simulink model "Simulator_Blockset"  (R2017b)
settings: Solver=VariableStepAuto  StartTime=0.0  StopTime=300  RelTol=1e-3  EnableMultiTasking=on
InitFcn:
  | Simulator_Init;
StopFcn:
  | % xia_out
values from neighbouring files (symbols this model uses):
  CC0 = 0    [Simulator_Init.m]
  CC_alpha = 0    [Simulator_Init.m]
  CC_beta = num(8,1)    [Simulator_Init.m]    (also in lat_eig.m = STB_LATin.DRVs.CC_beta)
  CC_dr = num(8,13)    [Simulator_Init.m]
  CC_p = num(8,4)    [Simulator_Init.m]
  CC_q = 0    [Simulator_Init.m]
  CC_r = num(8,5)    [Simulator_Init.m]
  CD0 = num(11,2)    [Simulator_Init.m]    (also in VLM2FG.m = Results.state(1,1).STC.friction.CD0; lat_chr.m = FILE.M_SDRV.state(1,1).STC.CD-FILE.M_SDRV.state(1,1).STC.CDi)
  CD_alpha = num(5,2)    [Simulator_Init.m]    (also in long_eig.m = results.CD_alpha)
  CD_alpha_dot = num(5,8)    [Simulator_Init.m]    (also in long_eig.m = 0)
  CD_beta = 0    [Simulator_Init.m]
  CD_dr = 0    [Simulator_Init.m]
  CD_p = num(5,17)    [Simulator_Init.m]
  CD_q = num(5,12)    [Simulator_Init.m]    (also in long_eig.m = results.CD_Q)
  CD_r = 0    [Simulator_Init.m]
  CL0 = num(11,1)    [Simulator_Init.m]
  CL_alpha = num(5,1)    [Simulator_Init.m]    (also in long_eig.m = results.CL_alpha; long_gfix.m = Mfile(i).M_SDRV.CL_alpha)
  CL_alpha_dot = num(5,7)    [Simulator_Init.m]    (also in long_eig.m = 0)
  CL_beta = num(5,16)    [Simulator_Init.m]
  CL_p = 0    [Simulator_Init.m]
  CL_q = num(5,10)    [Simulator_Init.m]    (also in long_eig.m = results.CL_Q)
  CL_r = 0    [Simulator_Init.m]
  Clm0 = 0    [Simulator_Init.m]
  Clm_alpha = 0    [Simulator_Init.m]
  Clm_beta = num(8,2)    [Simulator_Init.m]    (also in lat_eig.m = -0.074)
  Clm_da = num(8,11)    [Simulator_Init.m]
  Clm_dr = num(8,14)    [Simulator_Init.m]
  Clm_p = num(8,6)    [Simulator_Init.m]
  Clm_q = 0    [Simulator_Init.m]
  Clm_r = num(8,8)    [Simulator_Init.m]
  Cmm0 = 0    [Simulator_Init.m]
  Cmm_alpha = num(5,3)    [Simulator_Init.m]    (also in long_eig.m = results.CMm_alpha)
  Cmm_alpha_dot = num(5,9)    [Simulator_Init.m]    (also in long_eig.m = 0)
  Cmm_beta = 0    [Simulator_Init.m]
  Cmm_de = num(5,15)    [Simulator_Init.m]
  Cmm_p = num(8,19)    [Simulator_Init.m]
  Cmm_q = num(5,11)    [Simulator_Init.m]    (also in long_eig.m = results.CMm_Q)
  Cmm_r = 0    [Simulator_Init.m]
  Cnm0 = 0    [Simulator_Init.m]
  Cnm_alpha = 0    [Simulator_Init.m]
  Cnm_beta = num(8,3)    [Simulator_Init.m]    (also in lat_eig.m = 0.0701)
  Cnm_dr = num(8,15)    [Simulator_Init.m]
  Cnm_p = num(8,7)    [Simulator_Init.m]
  Cnm_q = 0    [Simulator_Init.m]
  Cnm_r = num(8,9)    [Simulator_Init.m]
  Engine = Ctrl.ENG    [Simulator_Init.m]
  F = double(F)    [PHD_paracamber.m]
  q = 0.5*state.rho*state.AS^2    [coeff_create3.m]    (also in coeff_hinge.m; lat_eig.m = 0.5*rho*V^2; long_eig.m = 0.5*rho*V^2; long_gfix.m = .5*allstate.rho*allstate.AS0(j)^2)
  uaero0 = [0 0 0 0]    [Simulator_Init.m]
undefined symbols (not defined in the file or in its folder): Earth, Light, MIL, model, WGS84
libraries: aerolibfltsims x3, aerolibadynsys x2, aerolibwind2 x2, aerolibanimutils x2, aerolibconvert2 x2, shared6dof x1, instrumentlib x1, sharedutil x1, aerolibasang x1, simulink_extras x1, aerolibatmos2 x1, aerolibobsolete x1
CloseFcn:
  | clear all;
settings Model: Creator=mc  LastModifiedBy=SONG
settings DataIOCC: LimitDataPoints=on  SaveFormat=Array
settings OptimizationCC: LifeSpan=inf
settings DebuggingCC: SolverPrmCheckMsg=warning  AllowSymbolicDim=off  SFUnexpectedBacktrackingDiag=warning  SFNoUnconditionalDefaultTransitionDiag=warning  SFExecutionAtInitializationDiag=none
settings HardwareCC: ProdBitPerPointer=32  ProdBitPerSizeT=32  ProdBitPerPtrDiffT=32  ProdLargestAtomicFloat=None  ProdIntDivRoundTo=Undefined  ProdEndianess=Unspecified  ProdWordSize=32  ProdHWDeviceType=32-bit Generic
settings ModelReferenceCC: PropagateSignalLabelsOutOfModel=off
settings CodeAppCC: StateflowObjectComments=on
settings GRTTargetCC: TargetLangStandard=C89/C90 (ANSI)  GeneratePreprocessorConditionals=Disable all
settings ConfigComp: CovMetricSettings=dw  CovHtmlReporting=on  CovSaveCumulativeToWorkspaceVar=on  CovSaveSingleToWorkspaceVar=on  CovExternalEMLEnable=off  CovSFcnEnable=off

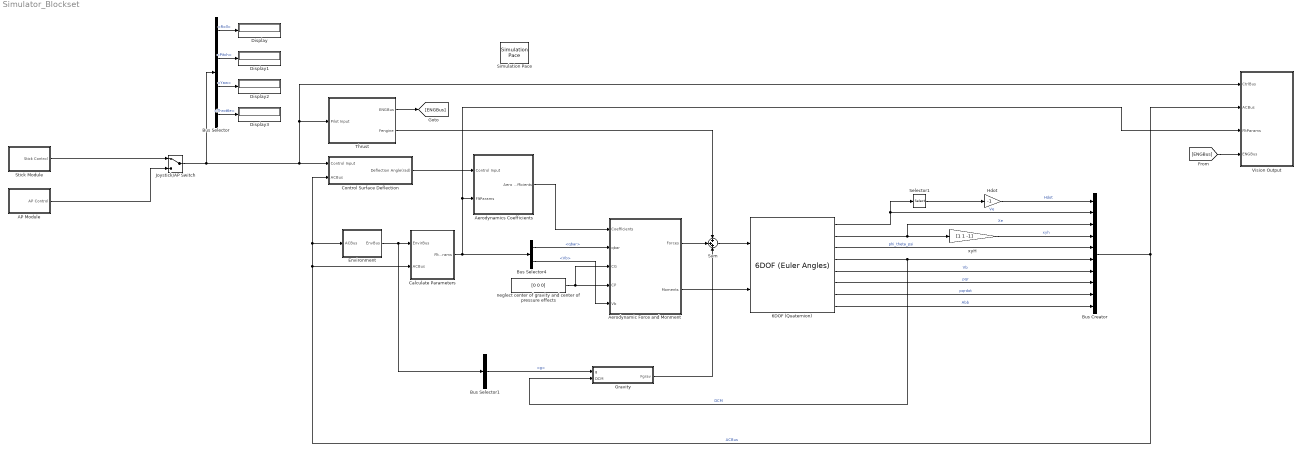
== system Simulator_Blockset ==
  6DOF (Quaternion) : shared6dof/6DOF (Euler Angles)  units=Metric (MKS)  mtype=Fixed  rep=Quaternion  xme_0=xme_0  Vm_0=[model.init.U model.init.V model.init.W]  eul_0=[model.init.roll, model.init.pitch, model.init.yaw]  pm_0=[model.init.P, model.init.Q, model.init.R]  mass_0=model.mass  mass_e=0  mass_f=0  inertia=[model.Ix -model.Ixy -model.Ixz; -model.Iyx model.Iy -model.Iyz; -model.Izx -model.Izy model.Iz]  inertia_e=eye(3)  inertia_f=eye(3)  k_quat=1.0  vre_flag=on  abi_flag=off
      settings: SourceProductBaseCode=AE
  AP Module : Subsystem
  Aerodynamic Force and Monment : Subsystem
  Aerodynamics Coefficients : Subsystem
  Bus Creator : BusCreator  Inputs=10
  Bus Selector : BusSelector  OutputSignals=Roll,Pitch,Yaw,Throttle
  Bus Selector1 : BusSelector  OutputSignals=g
  Bus Selector4 : BusSelector  OutputSignals=qbar,Vb
  Calculate Parameters : Subsystem
  Control Surface Deflection : Subsystem  mask{PitchUp_Lim=20, PitchDown_Lim=10, Roll_Lim=20, Yaw_Lim=20}
      mask prompts: PitchUp_Lim "Pitch Up Limit (Deg)"; PitchDown_Lim "Pitch Down Limit (Deg)"; Roll_Lim "Roll Limit (Deg)"; Yaw_Lim "Yaw Limit (Deg)"
      mask DialogControl ParameterGroupVar Prompt: Deflection Limits
  Display{,1..3} (4 alike) : Display
  Environment : Subsystem
  "Gravity " : Subsystem
  Hdot : Gain  Gain=-1  SaturateOnIntegerOverflow=on  OutDataTypeStr=Inherit: Same as input  ParamDataTypeStr=Inherit: Same as input
  Joystick/AP Switch : ManualSwitch
  Selector1 : Selector  IndexMode=Zero-based  InputPortWidth=3  IndexOptions=Index vector (dialog)  Indices=2  OutputSizes=1
  Simulation Pace : aerolibanimutils/Simulation Pace  SimulationPace=1  SleepMode=MATLAB Thread  OutputPaceError=off  SampleTime=1/50
      settings: AttributesFormatString=%<SimulationPace> sec/sec
  Stick Module : Subsystem
  Sum : Sum  Inputs=+++  SaturateOnIntegerOverflow=on  InputSameDT=on  OutDataTypeStr=Inherit: Same as first input
  Thrust : Subsystem
  Vision Output : Subsystem
  neglect center of gravity and center of pressure effects : Constant  Value=[0 0 0]
  xyH : Gain  Gain=[1 1 -1]  SaturateOnIntegerOverflow=on  OutDataTypeStr=Inherit: Same as input  ParamDataTypeStr=Inherit: Same as input
  wires:
  Hdot/1 -> Bus Creator/1  "Hdot"
  xyH/1 -> Bus Creator/4  "xyh"
  6DOF (Quaternion)/6 -> Bus Creator/8  "pqr"
  6DOF (Quaternion)/5 -> Bus Creator/7  "Vb"
  Aerodynamics Coefficients/1(Aero Coefficients) -> Aerodynamic Force and Monment/1(Coefficients)
  6DOF (Quaternion)/1 -> Selector1/1, Bus Creator/2  "Ve"
  Selector1/1 -> Hdot/1
  Environment/1(EnvBus) -> Bus Selector1/1, Calculate Parameters/1(EnvirBus)
  neglect center of gravity and center of pressure effects/1 -> Aerodynamic Force and Monment/3(CG), Aerodynamic Force and Monment/4(CP)
  Aerodynamic Force and Monment/2(Moments) -> 6DOF (Quaternion)/2
  6DOF (Quaternion)/7 -> Bus Creator/9  "pqrdot"
  6DOF (Quaternion)/3 -> Bus Creator/5  "phi_theta_psi"
  6DOF (Quaternion)/4 -> "Gravity "/2(DCM), Bus Creator/6  "DCM"
  6DOF (Quaternion)/2 -> Bus Creator/3, xyH/1  "Xe"
  Bus Selector4/1 -> Aerodynamic Force and Monment/2(qbar)  "<qbar>"
  Sum/1 -> 6DOF (Quaternion)/1
  "Gravity "/1(Fgrav) -> Sum/3
  Aerodynamic Force and Monment/1(Forces) -> Sum/2
  Bus Creator/1 -> Environment/1(ACBus), Control Surface Deflection/2(ACBus), Calculate Parameters/2(ACBus), Vision Output/2(ACBus)  "ACBus"
  Thrust/2(Fengine) -> Sum/1
  Calculate Parameters/1(FltParams) -> Vision Output/3(FltParams), Aerodynamics Coefficients/2(FltParams), Bus Selector4/1
  Bus Selector4/2 -> Aerodynamic Force and Monment/5(Vb)  "<Vb>"
  Bus Selector1/1 -> "Gravity "/1(g)  "<g>"
  Control Surface Deflection/1(Deflection Angle(rad)) -> Aerodynamics Coefficients/1(Control Input)
  Joystick/AP Switch/1 -> Bus Selector/1, Vision Output/1(CtrlBus), Thrust/1(Pilot Input), Control Surface Deflection/1(Control Input)
  Stick Module/1(Stick Control) -> Joystick/AP Switch/1
  6DOF (Quaternion)/8 -> Bus Creator/10  "Abb"
  AP Module/1(AP Control) -> Joystick/AP Switch/2
  Thrust/1(ENGBus) -> [ENGBus]
  [ENGBus] -> Vision Output/4(ENGBus)
  Bus Selector/4 -> Display3/1  "<Throttle>"
  Bus Selector/2 -> Display1/1  "<Pitch>"
  Bus Selector/1 -> Display/1  "<Roll>"
  Bus Selector/3 -> Display2/1  "<Yaw>"

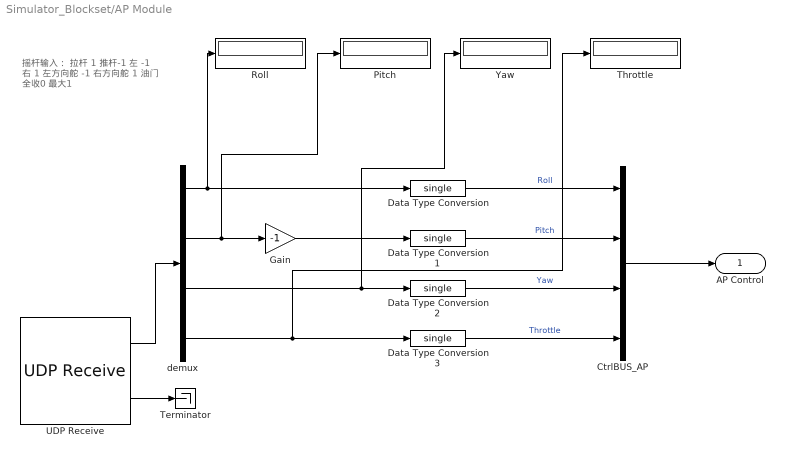
== system Simulator_Blockset/AP Module ==
  note: 摇杆输入：
      | 拉杆 1   推杆-1
      | 左   -1	右 1
      | 左方向舵 -1	右方向舵 1
      | 油门 全收0	最大1
  "CtrlBUS_AP " : BusCreator  Inputs=4
  Data Type Conversion{,1..3} (4 alike) : DataTypeConversion  OutDataTypeStr=single
  Gain : Gain  Gain=-1
  "Pitch " : Display
  Roll : Display
  Terminator : Terminator
  Throttle : Display
  UDP Receive : instrumentlib/UDP Receive  Host=127.0.0.1  Port=5500  LocalPort=49000  DataSize="[1  4]"  EnableBlockingMode=off  Timeout=10  SampleTime=-1  DataType=double  ByteOrder=BigEndian
      settings: SourceProductName=Instrument Control Toolbox
  Yaw : Display
  demux : Demux
  AP Control : Outport
  wires:
  demux/1 -> Roll/1, Data Type Conversion/1
  UDP Receive/2 -> Terminator/1
  UDP Receive/1 -> demux/1
  demux/3 -> Yaw/1, Data Type Conversion2/1
  demux/4 -> Throttle/1, Data Type Conversion3/1
  Data Type Conversion/1 -> "CtrlBUS_AP "/1  "Roll"
  Data Type Conversion1/1 -> "CtrlBUS_AP "/2  "Pitch"
  Data Type Conversion2/1 -> "CtrlBUS_AP "/3  "Yaw"
  Data Type Conversion3/1 -> "CtrlBUS_AP "/4  "Throttle"
  "CtrlBUS_AP "/1 -> AP Control/1
  demux/2 -> "Pitch "/1, Gain/1
  Gain/1 -> Data Type Conversion1/1

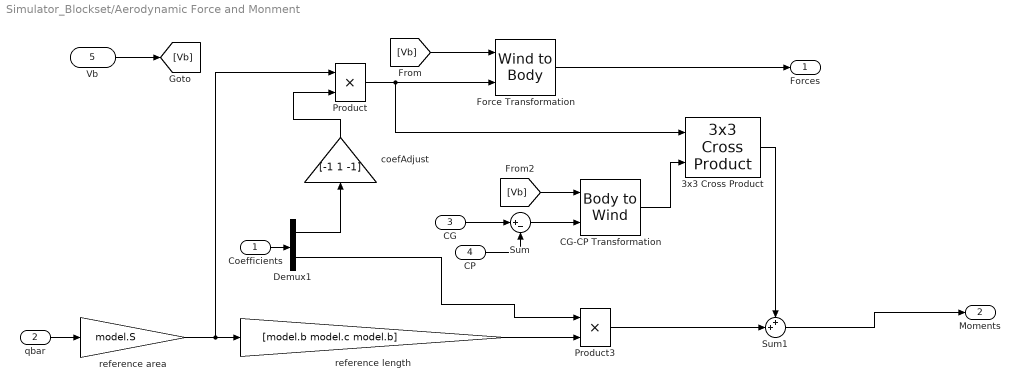
== system Simulator_Blockset/Aerodynamic Force and Monment ==
  Coefficients : Inport
  qbar : Inport  Port=2
  CG : Inport  Port=3
  CP : Inport  Port=4
  Vb : Inport  Port=5
  3x3 Cross Product : sharedutil/3x3 Cross Product
      settings: SourceProductBaseCode=AE
  CG-CP Transformation : aerolibadynsys/Body to Wind  SystemSampleTime=-1
      settings: SourceProductName=Aerospace Blockset  SourceProductBaseCode=AE
  Demux1 : Demux  Outputs=[3,3]
  Force Transformation : aerolibadynsys/Wind to Body  SystemSampleTime=-1
      settings: SourceProductName=Aerospace Blockset  SourceProductBaseCode=AE
  Product : Product  SaturateOnIntegerOverflow=on  InputSameDT=on  OutDataTypeStr=Inherit: Same as first input
  Product3 : Product  SaturateOnIntegerOverflow=on  InputSameDT=on  OutDataTypeStr=Inherit: Same as first input
  Sum : Sum  Inputs=|+-  SaturateOnIntegerOverflow=on
  Sum1 : Sum  Inputs=++|  SaturateOnIntegerOverflow=on  InputSameDT=on  OutDataTypeStr=Inherit: Same as first input
  coefAdjust : Gain  Gain=[-1 1 -1]
  reference area : Gain  Gain=model.S  SaturateOnIntegerOverflow=on  OutDataTypeStr=Inherit: Same as input  ParamDataTypeStr=Inherit: Same as input
  reference length : Gain  Gain=[model.b model.c model.b]  SaturateOnIntegerOverflow=on  OutDataTypeStr=Inherit: Same as input  ParamDataTypeStr=Inherit: Same as input
  Forces : Outport
  Moments : Outport  Port=2
  wires:
  3x3 Cross Product/1 -> Sum1/1
  reference length/1 -> Product3/2
  Coefficients/1 -> Demux1/1
  Demux1/2 -> Product3/1
  qbar/1 -> reference area/1
  reference area/1 -> reference length/1, Product/1
  Product3/1 -> Sum1/2
  Demux1/1 -> coefAdjust/1
  Product/1 -> Force Transformation/2, 3x3 Cross Product/1
  Force Transformation/1 -> Forces/1
  Vb/1 -> [Vb]
  [Vb] -> Force Transformation/1
  Sum1/1 -> Moments/1
  coefAdjust/1 -> Product/2
  CG/1 -> Sum/1
  CP/1 -> Sum/2
  Sum/1 -> CG-CP Transformation/2
  CG-CP Transformation/1 -> 3x3 Cross Product/2
  [Vb] -> CG-CP Transformation/1

== system Simulator_Blockset/Aerodynamics Coefficients ==
  Control Input : Inport
  FltParams : Inport  Port=2
  " Static Derivatives" : Subsystem
  Bus Selector1 : BusSelector  OutputSignals=alpha,beta
  Bus Selector2 : BusSelector  OutputSignals=V,pqr,alpha
  Control Derivatives : Subsystem
  Dynamic Derivatives : Subsystem
  Sum : Sum  Inputs=+++  SaturateOnIntegerOverflow=on
  Aero Coefficients : Outport
  wires:
  FltParams/1 -> Bus Selector1/1, Bus Selector2/1
  Bus Selector1/1 -> " Static Derivatives"/1(alpha)  "<alpha>"
  Bus Selector2/2 -> Dynamic Derivatives/2(p,q,r)  "<pqr>"
  Bus Selector2/1 -> Dynamic Derivatives/1(V)  "<V>"
  " Static Derivatives"/1(Coefficients) -> Sum/1
  Dynamic Derivatives/1(Coefficients) -> Sum/3
  Sum/1 -> Aero Coefficients/1
  Bus Selector1/2 -> " Static Derivatives"/2(beta)  "<beta>"
  Bus Selector2/3 -> Dynamic Derivatives/3(alpha)  "<alpha>"
  Control Derivatives/1(Coefficients) -> Sum/2
  Control Input/1 -> Control Derivatives/1(Control Input)

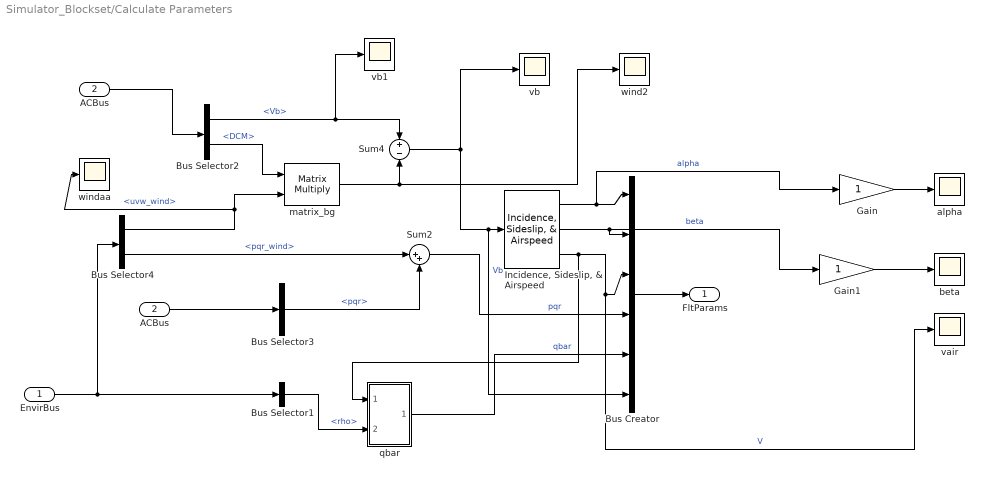
== system Simulator_Blockset/Calculate Parameters ==
  EnvirBus : Inport
  ACBus : Inport  Port=2
  "ACBus " : InportShadow  Port=2
  Bus Creator : BusCreator  Inputs=6
  Bus Selector1 : BusSelector  OutputSignals=rho
  Bus Selector2 : BusSelector  OutputSignals=Vb,DCM
  Bus Selector3 : BusSelector  OutputSignals=pqr
  Bus Selector4 : BusSelector  OutputSignals=signal3.uvw_wind,signal3.pqr_wind
  Gain : Gain
  Gain1 : Gain
  "Incidence, Sideslip, & Airspeed" : aerolibasang/Incidence, Sideslip, & Airspeed
      settings: SourceProductName=Aerospace Blockset
  Sum2 : Sum  Inputs=|++  SaturateOnIntegerOverflow=on  InputSameDT=on  OutDataTypeStr=Inherit: Same as first input
  Sum4 : Sum  Inputs=+-  SaturateOnIntegerOverflow=on  InputSameDT=on  OutDataTypeStr=Inherit: Same as first input
  alpha : Scope
  beta : Scope
  matrix_bg : Product  Multiplication=Matrix(*)
  qbar : Subsystem
  vair : Scope
  vb : Scope
  vb1 : Scope
  wind2 : Scope
  windaa : Scope
  FltParams : Outport
  wires:
  "Incidence, Sideslip, & Airspeed"/3 -> qbar/1(V_air), vair/1, Bus Creator/3  "V"
  "Incidence, Sideslip, & Airspeed"/2 -> Gain1/1, Bus Creator/2  "beta"
  "Incidence, Sideslip, & Airspeed"/1 -> Bus Creator/1, Gain/1  "alpha"
  ACBus/1 -> Bus Selector3/1
  Bus Creator/1 -> FltParams/1
  "ACBus "/1 -> Bus Selector2/1
  Gain/1 -> alpha/1
  Gain1/1 -> beta/1
  Bus Selector2/1 -> vb1/1, Sum4/1  "<Vb>"
  Sum4/1 -> Bus Creator/6, "Incidence, Sideslip, & Airspeed"/1, vb/1  "Vb"
  Bus Selector4/2 -> Sum2/1  "<pqr_wind>"
  Bus Selector3/1 -> Sum2/2  "<pqr>"
  Sum2/1 -> Bus Creator/4  "pqr"
  EnvirBus/1 -> Bus Selector4/1, Bus Selector1/1
  Bus Selector2/2 -> matrix_bg/1  "<DCM>"
  Bus Selector4/1 -> matrix_bg/2, windaa/1  "<uvw_wind>"
  matrix_bg/1 -> wind2/1, Sum4/2
  Bus Selector1/1 -> qbar/2(rho)  "<rho>"
  qbar/1(qbar) -> Bus Creator/5  "qbar"

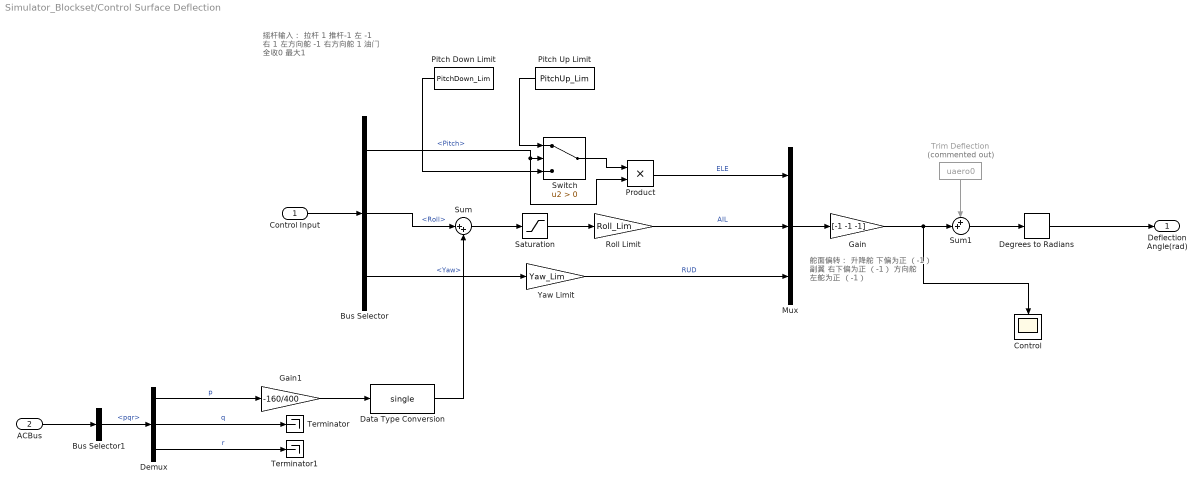
== system Simulator_Blockset/Control Surface Deflection ==
  note: 摇杆输入：
      | 拉杆 1   推杆-1
      | 左   -1	右 1
      | 左方向舵 -1	右方向舵 1
      | 油门 全收0	最大1
  note: 舵面偏转：
      | 升降舵	下偏为正	（-1）
      | 副翼	右下偏为正	（-1）
      | 方向舵	左舵为正	（-1）
  Control Input : Inport
  ACBus : Inport  Port=2
  Bus Selector : BusSelector  OutputSignals=Pitch,Roll,Yaw
  Bus Selector1 : BusSelector  OutputSignals=pqr
  Control : Scope
  Data Type Conversion : DataTypeConversion  OutDataTypeStr=single
  Degrees to Radians : simulink_extras/Transformations/Degrees to Radians
  Demux : Demux  Outputs=3
  Gain : Gain  Gain=[-1 -1 -1]
  Gain1 : Gain  Gain=-160/400
  Mux : Mux  Inputs=3
  Pitch Down Limit : Constant  Value=PitchDown_Lim  OutDataTypeStr=single
  Pitch Up Limit : Constant  Value=PitchUp_Lim  OutDataTypeStr=single
  Product : Product
  Roll Limit : Gain  Gain=Roll_Lim
  Saturation : Saturate  UpperLimit=1  LowerLimit=-1
  Sum : Sum  Inputs=|++
  Sum1 : Sum  Inputs=++|  SaturateOnIntegerOverflow=on  InputSameDT=on  OutDataTypeStr=Inherit: Same as first input
  Switch : Switch  Criteria=u2 > Threshold
  Terminator : Terminator
  Terminator1 : Terminator
  Trim Deflection : Constant  Commented=on  Value=uaero0
  Yaw Limit : Gain  Gain=Yaw_Lim
  Deflection Angle(rad) : Outport
  wires:
  Mux/1 -> Gain/1
  Sum1/1 -> Degrees to Radians/1
  Trim Deflection/1 -> Sum1/1
  Roll Limit/1 -> Mux/2  "AIL"
  Pitch Up Limit/1 -> Switch/1
  Pitch Down Limit/1 -> Switch/3
  Switch/1 -> Product/1
  Product/1 -> Mux/1  "ELE"
  Yaw Limit/1 -> Mux/3  "RUD"
  Degrees to Radians/1 -> Deflection Angle(rad)/1
  Gain/1 -> Control/1, Sum1/2
  Bus Selector/1 -> Product/2, Switch/2  "<Pitch>"
  Bus Selector/2 -> Sum/1  "<Roll>"
  Bus Selector/3 -> Yaw Limit/1  "<Yaw>"
  Control Input/1 -> Bus Selector/1
  ACBus/1 -> Bus Selector1/1
  Bus Selector1/1 -> Demux/1  "<pqr>"
  Demux/3 -> Terminator1/1  "r"
  Demux/2 -> Terminator/1  "q"
  Demux/1 -> Gain1/1  "p"
  Sum/1 -> Saturation/1
  Gain1/1 -> Data Type Conversion/1
  Data Type Conversion/1 -> Sum/2
  Saturation/1 -> Roll Limit/1

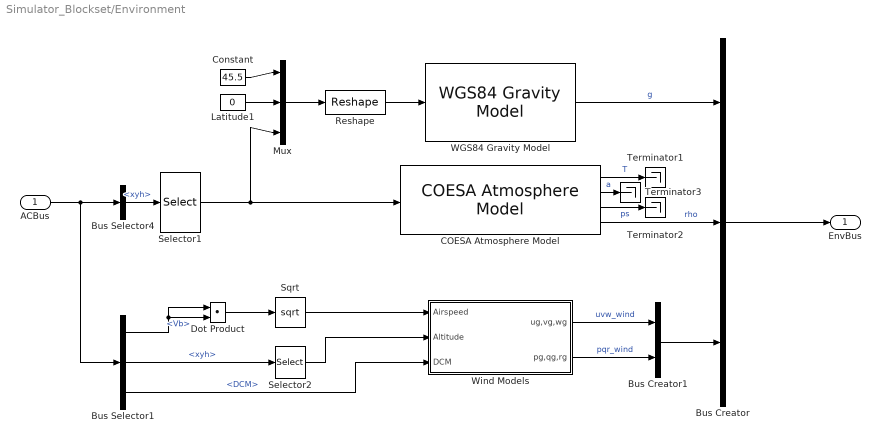
== system Simulator_Blockset/Environment ==
  ACBus : Inport
  Bus Creator : BusCreator  Inputs=3
  Bus Creator1 : BusCreator  Inputs=2
  Bus Selector1 : BusSelector  OutputSignals=Vb,xyh,DCM
  Bus Selector4 : BusSelector  OutputSignals=xyh
  COESA Atmosphere Model : aerolibatmos2/COESA Atmosphere Model  units=Metric (MKS)  spec=1976 COESA-extended U.S. Standard Atmosphere  model=Profile  profile_var=High temperature  profile_percent=1%  profile_alt=5 km (16404 ft)  envelope_var=High temperature  envelope_percent=1%  action=Warning
  Constant : Constant  Value=45.5
  Dot Product : DotProduct  OutDataTypeStr=double  InputSameDT=on
  Latitude1 : Constant  Value=0
  Mux : Mux  Inputs=3
  Reshape : Reshape  OutputDimensionality=Row vector (2-D)
  Selector1 : Selector  IndexMode=Zero-based  InputPortWidth=3  IndexOptions=Index vector (dialog)  Indices=2  OutputSizes=1
  Selector2 : Selector  IndexMode=Zero-based  InputPortWidth=3  IndexOptions=Index vector (dialog)  Indices=2  OutputSizes=1
  Sqrt : Sqrt  SaturateOnIntegerOverflow=on
  Terminator1 : Terminator
  Terminator2 : Terminator
  Terminator3 : Terminator
  "WGS84 Gravity Model " : aerolibobsolete/WGS84 Gravity Model   model=WGS84 Taylor Series  units=Metric (MKS)  no_atmos=on  precessing=on  jd_loc=off  month=October  day=10  year=2004  no_centrifugal=on  action=None
      settings: SourceProductName=Aerospace Blockset  SourceProductBaseCode=AE
  Wind Models : Subsystem
  EnvBus : Outport
  wires:
  Bus Selector4/1 -> Selector1/1  "<xyh>"
  ACBus/1 -> Bus Selector1/1, Bus Selector4/1
  Bus Creator/1 -> EnvBus/1
  COESA Atmosphere Model/2 -> Terminator3/1  "a"
  COESA Atmosphere Model/3 -> Terminator2/1  "ps"
  COESA Atmosphere Model/1 -> Terminator1/1  "T"
  COESA Atmosphere Model/4 -> Bus Creator/2  "rho"
  Selector1/1 -> COESA Atmosphere Model/1, Mux/3
  Constant/1 -> Mux/1
  Latitude1/1 -> Mux/2
  Mux/1 -> Reshape/1
  "WGS84 Gravity Model "/1 -> Bus Creator/1  "g"
  Reshape/1 -> "WGS84 Gravity Model "/1
  Bus Selector1/1 -> Dot Product/1, Dot Product/2  "<Vb>"
  Dot Product/1 -> Sqrt/1
  Sqrt/1 -> Wind Models/1(Airspeed)
  Bus Selector1/2 -> Selector2/1  "<xyh>"
  Selector2/1 -> Wind Models/2(Altitude)
  Bus Selector1/3 -> Wind Models/3(DCM)  "<DCM>"
  Wind Models/1(ug,vg,wg) -> Bus Creator1/1  "uvw_wind"
  Wind Models/2(pg,qg,rg) -> Bus Creator1/2  "pqr_wind"
  Bus Creator1/1 -> Bus Creator/3

== system Simulator_Blockset/Gravity  ==
  g : Inport
  DCM : Inport  Port=2
  Gravity in Earth Axes : Gain  Gain=model.mass  SaturateOnIntegerOverflow=on  OutDataTypeStr=Inherit: Same as input  ParamDataTypeStr=Inherit: Same as input
  Inertial to Body : Product  Multiplication=Matrix(*)  SaturateOnIntegerOverflow=on  InputSameDT=on  OutDataTypeStr=Inherit: Same as first input
  Reshape : Reshape  OutputDimensionality=Column vector (2-D)
  Reshape1 : Reshape
  Fgrav : Outport
  wires:
  Reshape1/1 -> Fgrav/1
  Reshape/1 -> Inertial to Body/2
  Gravity in Earth Axes/1 -> Reshape/1
  DCM/1 -> Inertial to Body/1
  g/1 -> Gravity in Earth Axes/1
  Inertial to Body/1 -> Reshape1/1

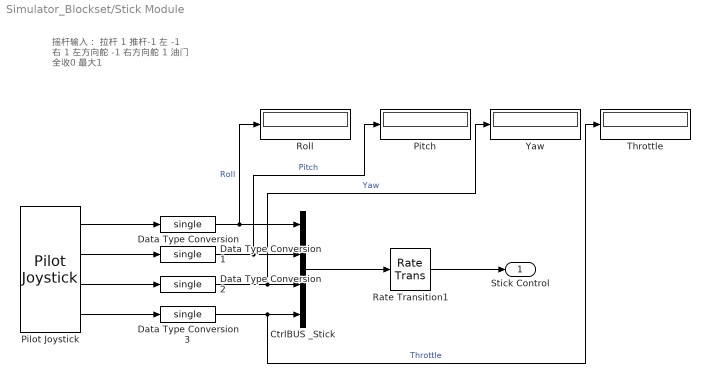
== system Simulator_Blockset/Stick Module ==
  note: 摇杆输入：
      | 拉杆 1   推杆-1
      | 左   -1	右 1
      | 左方向舵 -1	右方向舵 1
      | 油门 全收0	最大1
  CtrlBUS _Stick : BusCreator  Inputs=4
  Data Type Conversion{,1..3} (4 alike) : DataTypeConversion  OutDataTypeStr=single
  Pilot Joystick : aerolibanimutils/Pilot Joystick  JoystickID=Joystick1  OutputConfiguration=FourAxis  SampleTime=1/100
  Pitch : Display
  Rate Transition1 : RateTransition  OutPortSampleTime=0
  Roll : Display
  Throttle : Display
  Yaw : Display
  Stick Control : Outport
  wires:
  Pilot Joystick/1 -> Data Type Conversion/1
  CtrlBUS _Stick/1 -> Rate Transition1/1
  Rate Transition1/1 -> Stick Control/1
  Data Type Conversion/1 -> Roll/1, CtrlBUS _Stick/1  "Roll"
  Pilot Joystick/2 -> Data Type Conversion1/1
  Pilot Joystick/4 -> Data Type Conversion3/1
  Pilot Joystick/3 -> Data Type Conversion2/1
  Data Type Conversion1/1 -> Pitch/1, CtrlBUS _Stick/2  "Pitch"
  Data Type Conversion2/1 -> Yaw/1, CtrlBUS _Stick/3  "Yaw"
  Data Type Conversion3/1 -> Throttle/1, CtrlBUS _Stick/4  "Throttle"

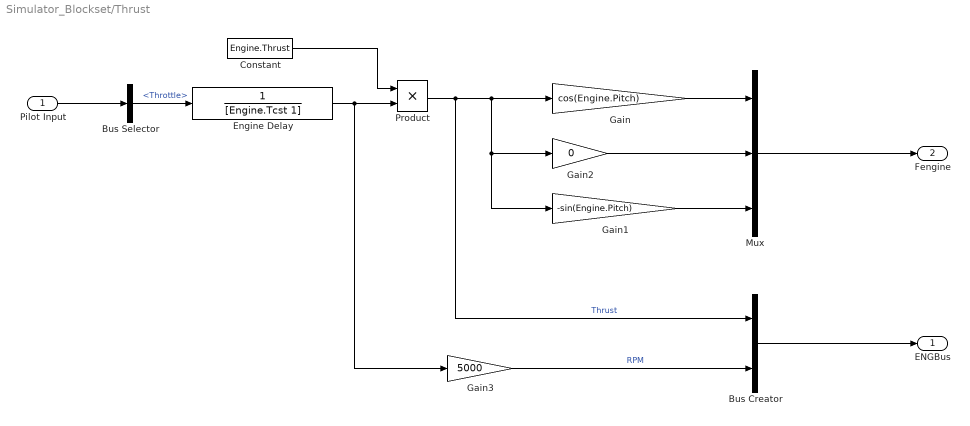
== system Simulator_Blockset/Thrust ==
  Pilot Input : Inport
  Bus Creator : BusCreator  Inputs=2
  Bus Selector : BusSelector  OutputSignals=Throttle
  Constant : Constant  Value=Engine.Thrust
  Engine Delay : TransferFcn  Denominator=[Engine.Tcst 1]
  Gain : Gain  Gain=cos(Engine.Pitch)
  Gain1 : Gain  Gain=-sin(Engine.Pitch)
  Gain2 : Gain  Gain=0
  Gain3 : Gain  Gain=5000
  Mux : Mux  Inputs=3
  Product : Product
  ENGBus : Outport
  Fengine : Outport  Port=2
  wires:
  Pilot Input/1 -> Bus Selector/1
  Mux/1 -> Fengine/1
  Constant/1 -> Product/1
  Gain2/1 -> Mux/2
  Gain/1 -> Mux/1
  Gain1/1 -> Mux/3
  Bus Creator/1 -> ENGBus/1
  Product/1 -> Bus Creator/1, Gain2/1, Gain1/1, Gain/1  "Thrust"
  Engine Delay/1 -> Gain3/1, Product/2
  Bus Selector/1 -> Engine Delay/1  "<Throttle>"
  Gain3/1 -> Bus Creator/2  "RPM"

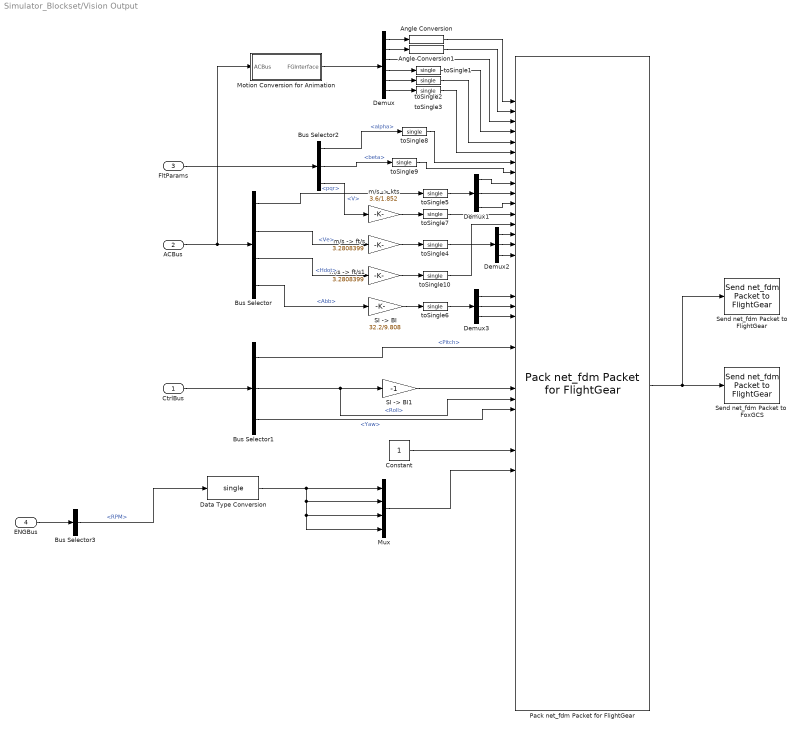
== system Simulator_Blockset/Vision Output ==
  CtrlBus : Inport
  ACBus : Inport  Port=2
  FltParams : Inport  Port=3
  ENGBus : Inport  Port=4
  Angle Conversion : aerolibconvert2/Angle Conversion  IU=deg  OU=rad
  Angle Conversion1 : aerolibconvert2/Angle Conversion  IU=deg  OU=rad
  Bus Selector : BusSelector  OutputSignals=pqr,Ve,Hdot,Abb
  Bus Selector1 : BusSelector  OutputSignals=Pitch,Roll,Yaw
  Bus Selector2 : BusSelector  OutputSignals=alpha,beta,V
  Bus Selector3 : BusSelector  OutputSignals=RPM
  Constant : Constant  OutDataTypeStr=uint32
  Data Type Conversion : DataTypeConversion  OutDataTypeStr=single
  Demux : Demux  Outputs=6
  Demux1 : Demux  Outputs=3
  Demux2 : Demux  Outputs=3
  Demux3 : Demux  Outputs=3
  Motion Conversion for Animation : Subsystem
      mask Display:
      | port_label('input',1,'ACBus')
      | port_label('output',1,'\lambda,L,h,\phi,\theta,\psi','texmode','on')
  Mux : Mux
  Pack net_fdm Packet for FlightGear : aerolibfltsims/Pack net_fdm Packet for FlightGear  FlightGearVersion=v2017.1  ShowPositionAttitudeInputs=on  ShowVelocityAccelerationInputs=on  ShowControlSurfacePositionInputs=on  ShowEngineFuelInputs=on  ShowLandingGearInputs=on  ShowEnvironmentInputs=on  SampleTime=1/100
      settings: SourceProductName=Aerospace Blockset  SourceProductBaseCode=AE
  "SI -> BI" : Gain  Gain=32.2/9.808
  "SI -> BI1" : Gain  Gain=-1
  Send net_fdm Packet to  FoxGCS : aerolibfltsims/Send net_fdm Packet to FlightGear  DestinationIpAddress=127.0.0.1  DestinationPort=49005  LocalIpPort=-1  varLen=off  SampleTime=1/50
      settings: SourceProductName=Aerospace Blockset  SourceProductBaseCode=AE
  Send net_fdm Packet to FlightGear : aerolibfltsims/Send net_fdm Packet to FlightGear  DestinationIpAddress=127.0.0.1  DestinationPort=5502  LocalIpPort=-1  varLen=off  SampleTime=1/100
      settings: SourceProductName=Aerospace Blockset  SourceProductBaseCode=AE
  "m/s -> ft/s" : Gain  Gain=3.2808399
  "m/s -> ft/s1" : Gain  Gain=3.2808399
  "m/s -> kts" : Gain  Gain=3.6/1.852
  toSingle{1..10} (10 alike) : DataTypeConversion  OutDataTypeStr=single
  wires:
  Bus Selector2/2 -> toSingle9/1  "<beta>"
  toSingle1/1 -> Pack net_fdm Packet for FlightGear/4
  Demux/5 -> toSingle2/1
  toSingle3/1 -> Pack net_fdm Packet for FlightGear/6
  Motion Conversion for Animation/1(FGInterface) -> Demux/1
  Demux/3 -> Pack net_fdm Packet for FlightGear/3
  Demux/6 -> toSingle3/1
  Demux/2 -> Angle Conversion1/1
  Angle Conversion1/1 -> Pack net_fdm Packet for FlightGear/2
  Demux/1 -> Angle Conversion/1
  Demux/4 -> toSingle1/1
  Pack net_fdm Packet for FlightGear/1 -> Send net_fdm Packet to FlightGear/1, Send net_fdm Packet to  FoxGCS/1
  toSingle2/1 -> Pack net_fdm Packet for FlightGear/5
  Angle Conversion/1 -> Pack net_fdm Packet for FlightGear/1
  Demux1/1 -> Pack net_fdm Packet for FlightGear/9
  Demux1/2 -> Pack net_fdm Packet for FlightGear/10
  Demux1/3 -> Pack net_fdm Packet for FlightGear/11
  Demux2/2 -> Pack net_fdm Packet for FlightGear/15
  Demux2/3 -> Pack net_fdm Packet for FlightGear/16
  Demux2/1 -> Pack net_fdm Packet for FlightGear/14
  "m/s -> ft/s"/1 -> toSingle4/1
  toSingle4/1 -> Demux2/1
  toSingle5/1 -> Demux1/1
  Demux3/2 -> Pack net_fdm Packet for FlightGear/21
  Demux3/3 -> Pack net_fdm Packet for FlightGear/22
  "SI -> BI"/1 -> toSingle6/1
  toSingle6/1 -> Demux3/1
  Demux3/1 -> Pack net_fdm Packet for FlightGear/20
  "m/s -> kts"/1 -> toSingle7/1
  Bus Selector2/3 -> "m/s -> kts"/1  "<V>"
  toSingle7/1 -> Pack net_fdm Packet for FlightGear/12
  toSingle9/1 -> Pack net_fdm Packet for FlightGear/8
  Bus Selector2/1 -> toSingle8/1  "<alpha>"
  toSingle8/1 -> Pack net_fdm Packet for FlightGear/7
  FltParams/1 -> Bus Selector2/1
  ACBus/1 -> Motion Conversion for Animation/1(ACBus), Bus Selector/1
  Bus Selector/2 -> "m/s -> ft/s"/1  "<Ve>"
  Bus Selector/1 -> toSingle5/1  "<pqr>"
  Bus Selector/3 -> "m/s -> ft/s1"/1  "<Hdot>"
  "m/s -> ft/s1"/1 -> toSingle10/1
  toSingle10/1 -> Pack net_fdm Packet for FlightGear/13
  Bus Selector/4 -> "SI -> BI"/1  "<Abb>"
  CtrlBus/1 -> Bus Selector1/1
  Bus Selector1/1 -> Pack net_fdm Packet for FlightGear/25  "<Pitch>"
  Bus Selector1/2 -> Pack net_fdm Packet for FlightGear/30, "SI -> BI1"/1  "<Roll>"
  "SI -> BI1"/1 -> Pack net_fdm Packet for FlightGear/29
  Bus Selector1/3 -> Pack net_fdm Packet for FlightGear/31  "<Yaw>"
  Constant/1 -> Pack net_fdm Packet for FlightGear/35
  ENGBus/1 -> Bus Selector3/1
  Mux/1 -> Pack net_fdm Packet for FlightGear/37
  Bus Selector3/1 -> Data Type Conversion/1  "<RPM>"
  Data Type Conversion/1 -> Mux/2, Mux/4, Mux/3, Mux/1

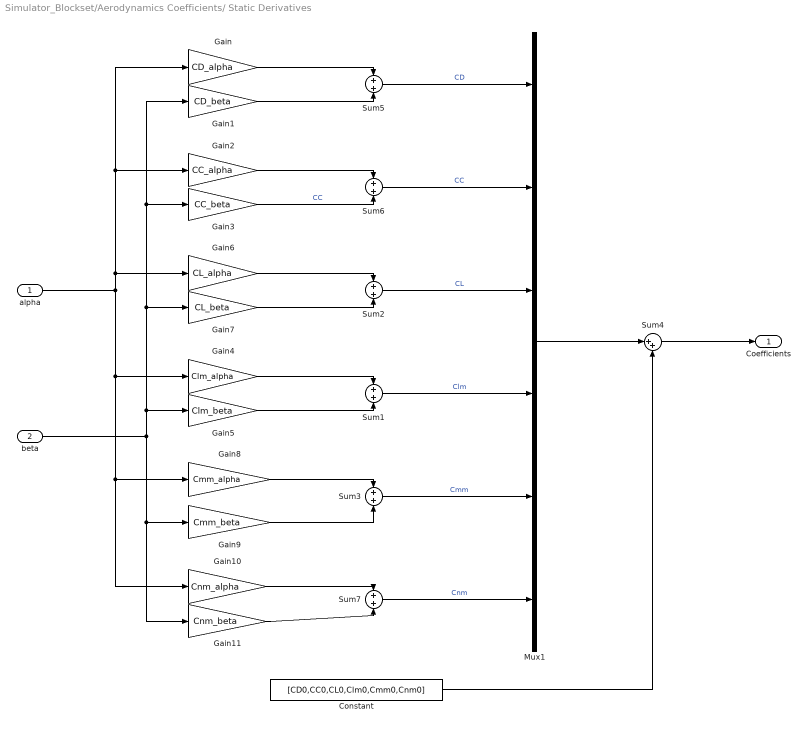
== system Simulator_Blockset/Aerodynamics Coefficients/ Static Derivatives ==
  alpha : Inport
  beta : Inport  Port=2
  Constant : Constant  Value=[CD0,CC0,CL0,Clm0,Cmm0,Cnm0]
  Gain : Gain  Gain=CD_alpha  SaturateOnIntegerOverflow=on  OutDataTypeStr=Inherit: Same as input  ParamDataTypeStr=Inherit: Same as input
  Gain1 : Gain  Gain=CD_beta  SaturateOnIntegerOverflow=on  OutDataTypeStr=Inherit: Same as input  ParamDataTypeStr=Inherit: Same as input
  Gain10 : Gain  Gain=Cnm_alpha  SaturateOnIntegerOverflow=on  OutDataTypeStr=Inherit: Same as input  ParamDataTypeStr=Inherit: Same as input
  Gain11 : Gain  Gain=Cnm_beta  SaturateOnIntegerOverflow=on  OutDataTypeStr=Inherit: Same as input  ParamDataTypeStr=Inherit: Same as input
  Gain2 : Gain  Gain=CC_alpha  SaturateOnIntegerOverflow=on  OutDataTypeStr=Inherit: Same as input  ParamDataTypeStr=Inherit: Same as input
  Gain3 : Gain  Gain=CC_beta  SaturateOnIntegerOverflow=on  OutDataTypeStr=Inherit: Same as input  ParamDataTypeStr=Inherit: Same as input
  Gain4 : Gain  Gain=Clm_alpha  SaturateOnIntegerOverflow=on  OutDataTypeStr=Inherit: Same as input  ParamDataTypeStr=Inherit: Same as input
  Gain5 : Gain  Gain=Clm_beta  SaturateOnIntegerOverflow=on  OutDataTypeStr=Inherit: Same as input  ParamDataTypeStr=Inherit: Same as input
  Gain6 : Gain  Gain=CL_alpha  SaturateOnIntegerOverflow=on  OutDataTypeStr=Inherit: Same as input  ParamDataTypeStr=Inherit: Same as input
  Gain7 : Gain  Gain=CL_beta  SaturateOnIntegerOverflow=on  OutDataTypeStr=Inherit: Same as input  ParamDataTypeStr=Inherit: Same as input
  Gain8 : Gain  Gain=Cmm_alpha  SaturateOnIntegerOverflow=on  OutDataTypeStr=Inherit: Same as input  ParamDataTypeStr=Inherit: Same as input
  Gain9 : Gain  Gain=Cmm_beta  SaturateOnIntegerOverflow=on  OutDataTypeStr=Inherit: Same as input  ParamDataTypeStr=Inherit: Same as input
  Mux1 : Mux  Inputs=6
  Sum{1..3,5..7} (6 alike) : Sum  SaturateOnIntegerOverflow=on
  Sum4 : Sum  Inputs=|++  SaturateOnIntegerOverflow=on
  Coefficients : Outport
  wires:
  beta/1 -> Gain3/1, Gain1/1, Gain7/1, Gain5/1, Gain9/1, Gain11/1
  alpha/1 -> Gain6/1, Gain2/1, Gain/1, Gain10/1, Gain8/1, Gain4/1
  Mux1/1 -> Sum4/1
  Sum4/1 -> Coefficients/1
  Constant/1 -> Sum4/2
  Gain/1 -> Sum5/1
  Sum5/1 -> Mux1/1  "CD"
  Gain1/1 -> Sum5/2
  Sum6/1 -> Mux1/2  "CC"
  Gain3/1 -> Sum6/2  "CC"
  Gain2/1 -> Sum6/1
  Gain6/1 -> Sum2/1
  Gain7/1 -> Sum2/2
  Sum2/1 -> Mux1/3  "CL"
  Gain4/1 -> Sum1/1
  Gain5/1 -> Sum1/2
  Gain8/1 -> Sum3/1
  Gain9/1 -> Sum3/2
  Gain10/1 -> Sum7/1
  Gain11/1 -> Sum7/2
  Sum7/1 -> Mux1/6  "Cnm"
  Sum1/1 -> Mux1/4  "Clm"
  Sum3/1 -> Mux1/5  "Cmm"

== system Simulator_Blockset/Aerodynamics Coefficients/Control Derivatives ==
  Control Input : Inport
  Aileron : Subsystem
  Elevator : Subsystem
  Rudder : Subsystem
  Sum : Sum  Inputs=+++  SaturateOnIntegerOverflow=on  InputSameDT=on  OutDataTypeStr=Inherit: Same as first input
  Coefficients : Outport
  wires:
  Sum/1 -> Coefficients/1
  Rudder/1(delCoeff) -> Sum/3
  Elevator/1(delCoeff) -> Sum/2
  Aileron/1(delCoeff) -> Sum/1
  Control Input/1 -> Aileron/1(Actuators), Elevator/1(Actuators), Rudder/1(Actuators)

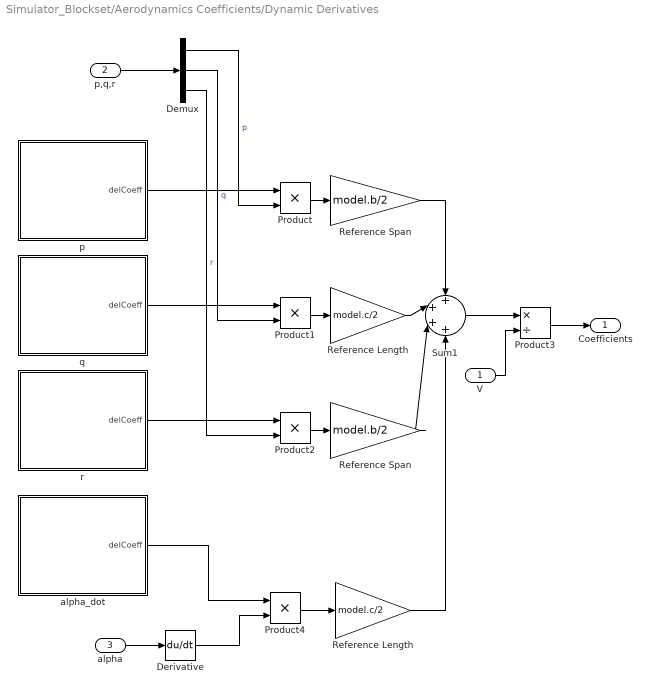
== system Simulator_Blockset/Aerodynamics Coefficients/Dynamic Derivatives ==
  V : Inport
  p,q,r : Inport  Port=2
  alpha : Inport  Port=3
  Demux : Demux  Outputs=3
  Derivative : Derivative
  Product{,1..2,4} (4 alike) : Product  SaturateOnIntegerOverflow=on  InputSameDT=on  OutDataTypeStr=Inherit: Same as first input
  Product3 : Product  Inputs=*/  SaturateOnIntegerOverflow=on  InputSameDT=on  OutDataTypeStr=Inherit: Same as first input
  Reference Length : Gain  Gain=model.c/2  SaturateOnIntegerOverflow=on  OutDataTypeStr=Inherit: Same as input  ParamDataTypeStr=Inherit: Same as input
  "Reference Length " : Gain  Gain=model.c/2  SaturateOnIntegerOverflow=on  OutDataTypeStr=Inherit: Same as input  ParamDataTypeStr=Inherit: Same as input
  Reference Span : Gain  Gain=model.b/2  SaturateOnIntegerOverflow=on  OutDataTypeStr=Inherit: Same as input  ParamDataTypeStr=Inherit: Same as input
  "Reference Span " : Gain  Gain=model.b/2  SaturateOnIntegerOverflow=on  OutDataTypeStr=Inherit: Same as input  ParamDataTypeStr=Inherit: Same as input
  Sum1 : Sum  Inputs=++++  SaturateOnIntegerOverflow=on  InputSameDT=on  OutDataTypeStr=Inherit: Same as first input
  alpha_dot : Subsystem
  p : Subsystem
  q : Subsystem
  r : Subsystem
  Coefficients : Outport
  wires:
  "Reference Span "/1 -> Sum1/3
  Reference Span/1 -> Sum1/1
  Reference Length/1 -> Sum1/2
  r/1(delCoeff) -> Product2/1
  Product/1 -> Reference Span/1
  Product2/1 -> "Reference Span "/1
  Product1/1 -> Reference Length/1
  Product3/1 -> Coefficients/1
  Sum1/1 -> Product3/1
  q/1(delCoeff) -> Product1/1
  p/1(delCoeff) -> Product/1
  Product4/1 -> "Reference Length "/1
  alpha_dot/1(delCoeff) -> Product4/1
  p,q,r/1 -> Demux/1
  V/1 -> Product3/2
  Demux/1 -> Product/2  "p"
  Demux/2 -> Product1/2  "q"
  Demux/3 -> Product2/2  "r"
  alpha/1 -> Derivative/1
  "Reference Length "/1 -> Sum1/4
  Derivative/1 -> Product4/2

== system Simulator_Blockset/Calculate Parameters/qbar ==
  V_air : Inport
  rho : Inport  Port=2
  Constant : Constant  Value=0.5
  Product : Product  Inputs=3
  Product1 : Product
  qbar : Outport
  wires:
  V_air/1 -> Product1/2, Product1/1
  rho/1 -> Product/1
  Product1/1 -> Product/3
  Product/1 -> qbar/1
  Constant/1 -> Product/2

== system Simulator_Blockset/Environment/Wind Models ==
  Airspeed : Inport
  Altitude : Inport  Port=2
  DCM : Inport  Port=3
  Discrete Wind Gust Model : aerolibwind2/Discrete Wind Gust Model  units=Metric (MKS)  Gx=off  Gy=off  Gz=off  t_0=0  d_m=[0.01 0.01 2*model.init.U]  v_m=[0.01 0.01 -10]
      settings: SourceProductName=Aerospace Blockset
  Dryden Wind Turbulence Model (Continuous (+q -r)) : aerolibwind2/Dryden Wind Turbulence Model  (Continuous (+q -r))  units=Metric (MKS)  spec=MIL-F-8785C  model=Continuous Dryden (+q -r)  W20=1  Wdeg=1  TurbProb=10^-2 - Light  L_high=1  Wingspan=10  ts=1  Seed=[1 1 1 1]  T_on=off
      settings: SourceProductName=Aerospace Blockset
  Sum : Sum  SaturateOnIntegerOverflow=on  InputSameDT=on  OutDataTypeStr=Inherit: Same as first input
  Vwind : Scope
  Vwind1 : Scope
  ug,vg,wg : Outport
  pg,qg,rg : Outport  Port=2
  wires:
  Sum/1 -> ug,vg,wg/1
  DCM/1 -> Dryden Wind Turbulence Model (Continuous (+q -r))/3
  Discrete Wind Gust Model/1 -> Sum/2, Vwind/1
  Airspeed/1 -> Discrete Wind Gust Model/1, Dryden Wind Turbulence Model (Continuous (+q -r))/2
  Altitude/1 -> Dryden Wind Turbulence Model (Continuous (+q -r))/1
  Dryden Wind Turbulence Model (Continuous (+q -r))/1 -> Sum/1, Vwind1/1
  Dryden Wind Turbulence Model (Continuous (+q -r))/2 -> pg,qg,rg/1

== system Simulator_Blockset/Vision Output/Motion Conversion for Animation ==
  ACBus : Inport
  Bus Selector : BusSelector  OutputSignals=phi_theta_psi
  Bus Selector1 : BusSelector  OutputSignals=Xe  OutputAsBus=on
  Constant : Constant  Value=0
  Flat Earth to LLA : aerolibtransform2/Flat Earth to LLA  units=Metric (MKS)  ptype=Earth (WGS84)  F=1/298.257223563  R=6378137  LL0=[37.6272 -122.3896]  psi=0
  Mux : Mux  Inputs=2
  Mux1 : Mux  Inputs=2
  Selector : Selector  IndexMode=Zero-based  InputPortWidth=2  IndexOptions=Index vector (dialog)  Indices=[1 0]  OutputSizes=1
  FGInterface : Outport
  wires:
  Selector/1 -> Mux/1
  ACBus/1 -> Bus Selector1/1, Bus Selector/1
  Bus Selector1/1 -> Flat Earth to LLA/1
  Flat Earth to LLA/1 -> Selector/1
  Flat Earth to LLA/2 -> Mux/2
  Mux/1 -> Mux1/1
  Bus Selector/1 -> Mux1/2  "<phi_theta_psi>"
  Constant/1 -> Flat Earth to LLA/2
  Mux1/1 -> FGInterface/1

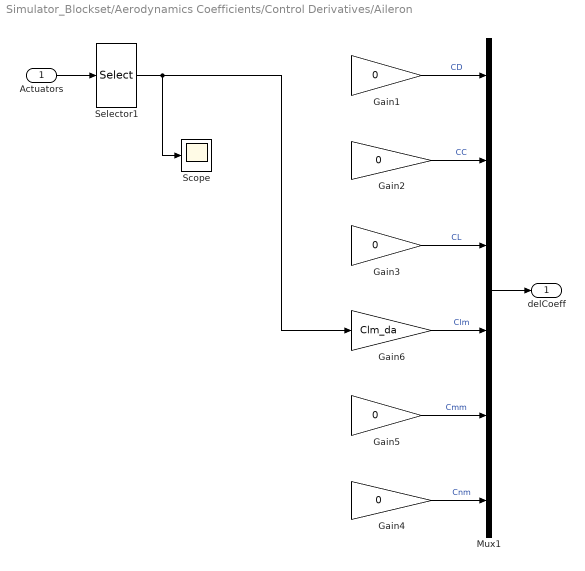
== system Simulator_Blockset/Aerodynamics Coefficients/Control Derivatives/Aileron ==
  Actuators : Inport
  Gain{1..5} (5 alike) : Gain  Gain=0  SaturateOnIntegerOverflow=on  OutDataTypeStr=Inherit: Same as input  ParamDataTypeStr=Inherit: Same as input
  Gain6 : Gain  Gain=Clm_da  SaturateOnIntegerOverflow=on  OutDataTypeStr=Inherit: Same as input  ParamDataTypeStr=Inherit: Same as input
  Mux1 : Mux  Inputs=6
  Scope : Scope
  Selector1 : Selector  InputPortWidth=3  IndexOptions=Index vector (dialog)  Indices=2  OutputSizes=1
  delCoeff : Outport
  wires:
  Gain4/1 -> Mux1/6  "Cnm"
  Gain5/1 -> Mux1/5  "Cmm"
  Gain3/1 -> Mux1/3  "CL"
  Gain2/1 -> Mux1/2  "CC"
  Mux1/1 -> delCoeff/1
  Actuators/1 -> Selector1/1
  Gain1/1 -> Mux1/1  "CD"
  Gain6/1 -> Mux1/4  "Clm"
  Selector1/1 -> Gain6/1, Scope/1

== system Simulator_Blockset/Aerodynamics Coefficients/Control Derivatives/Elevator ==
  Actuators : Inport
  Gain{1..5} (5 alike) : Gain  Gain=0  SaturateOnIntegerOverflow=on  OutDataTypeStr=Inherit: Same as input  ParamDataTypeStr=Inherit: Same as input
  Gain6 : Gain  Gain=Cmm_de  SaturateOnIntegerOverflow=on  OutDataTypeStr=Inherit: Same as input  ParamDataTypeStr=Inherit: Same as input
  Mux1 : Mux  Inputs=6
  Scope : Scope
  Selector1 : Selector  InputPortWidth=3  IndexOptions=Index vector (dialog)  Indices=1  OutputSizes=1
  delCoeff : Outport
  wires:
  Actuators/1 -> Selector1/1
  Mux1/1 -> delCoeff/1
  Gain1/1 -> Mux1/3  "CL"
  Gain5/1 -> Mux1/4  "Clm"
  Gain2/1 -> Mux1/2  "CC"
  Gain4/1 -> Mux1/1  "CD"
  Selector1/1 -> Gain6/1, Scope/1
  Gain6/1 -> Mux1/5  "Cmm"
  Gain3/1 -> Mux1/6  "Cnm"

== system Simulator_Blockset/Aerodynamics Coefficients/Control Derivatives/Rudder ==
  Actuators : Inport
  Gain1 : Gain  Gain=Clm_dr  SaturateOnIntegerOverflow=on  OutDataTypeStr=Inherit: Same as input  ParamDataTypeStr=Inherit: Same as input
  Gain2 : Gain  Gain=Cnm_dr  SaturateOnIntegerOverflow=on  OutDataTypeStr=Inherit: Same as input  ParamDataTypeStr=Inherit: Same as input
  Gain3 : Gain  Gain=0  SaturateOnIntegerOverflow=on  OutDataTypeStr=Inherit: Same as input  ParamDataTypeStr=Inherit: Same as input
  Gain4 : Gain  Gain=CC_dr  SaturateOnIntegerOverflow=on  OutDataTypeStr=Inherit: Same as input  ParamDataTypeStr=Inherit: Same as input
  Gain5 : Gain  Gain=CD_dr  SaturateOnIntegerOverflow=on  OutDataTypeStr=Inherit: Same as input  ParamDataTypeStr=Inherit: Same as input
  Gain6 : Gain  Gain=0  SaturateOnIntegerOverflow=on  OutDataTypeStr=Inherit: Same as input  ParamDataTypeStr=Inherit: Same as input
  Mux1 : Mux  Inputs=6
  Scope : Scope
  Selector1 : Selector  InputPortWidth=3  IndexOptions=Index vector (dialog)  Indices=3  OutputSizes=1
  delCoeff : Outport
  wires:
  Selector1/1 -> Scope/1, Gain5/1, Gain4/1, Gain3/1, Gain6/1, Gain2/1, Gain1/1
  Actuators/1 -> Selector1/1
  Mux1/1 -> delCoeff/1
  Gain2/1 -> Mux1/6  "Cnm"
  Gain1/1 -> Mux1/4  "Clm"
  Gain4/1 -> Mux1/2  "CC"
  Gain5/1 -> Mux1/1  "CD"
  Gain3/1 -> Mux1/3  "CL"
  Gain6/1 -> Mux1/5  "Cmm"

== system Simulator_Blockset/Aerodynamics Coefficients/Dynamic Derivatives/alpha_dot ==
  Constant : Constant  Value=CD_alpha_dot
  Constant1 : Constant  Value=0
  Constant2 : Constant  Value=0
  Constant3 : Constant  Value=Cmm_alpha_dot
  Constant4 : Constant  Value=0
  Constant5 : Constant  Value=CL_alpha_dot
  Mux1 : Mux  Inputs=6
  delCoeff : Outport
  wires:
  Mux1/1 -> delCoeff/1
  Constant/1 -> Mux1/1  "CD"
  Constant2/1 -> Mux1/4  "Clm"
  Constant4/1 -> Mux1/6  "Cnm"
  Constant1/1 -> Mux1/2  "CC"
  Constant3/1 -> Mux1/5  "Cmm"
  Constant5/1 -> Mux1/3  "CL"

== system Simulator_Blockset/Aerodynamics Coefficients/Dynamic Derivatives/p ==
  Constant1 : Constant  Value=CD_p
  Constant2 : Constant  Value=CC_p
  Constant3 : Constant  Value=Clm_p
  Constant4 : Constant  Value=Cnm_p
  Constant5 : Constant  Value=CL_p
  Constant6 : Constant  Value=Cmm_p
  Mux1 : Mux  Inputs=6
  delCoeff : Outport
  wires:
  Mux1/1 -> delCoeff/1
  Constant1/1 -> Mux1/1  "CD"
  Constant2/1 -> Mux1/2  "CC"
  Constant5/1 -> Mux1/3  "CL"
  Constant3/1 -> Mux1/4  "Clm"
  Constant6/1 -> Mux1/5  "Cmm"
  Constant4/1 -> Mux1/6  "Cnm"

== system Simulator_Blockset/Aerodynamics Coefficients/Dynamic Derivatives/q ==
  Constant1 : Constant  Value=CD_q
  Constant2 : Constant  Value=CC_q
  Constant3 : Constant  Value=Clm_q
  Constant4 : Constant  Value=Cnm_q
  Constant5 : Constant  Value=CL_q
  Constant6 : Constant  Value=Cmm_q
  Mux1 : Mux  Inputs=6
  delCoeff : Outport
  wires:
  Mux1/1 -> delCoeff/1
  Constant1/1 -> Mux1/1
  Constant2/1 -> Mux1/2
  Constant5/1 -> Mux1/3
  Constant3/1 -> Mux1/4
  Constant6/1 -> Mux1/5
  Constant4/1 -> Mux1/6

== system Simulator_Blockset/Aerodynamics Coefficients/Dynamic Derivatives/r ==
  Constant1 : Constant  Value=CD_r
  Constant2 : Constant  Value=CC_r
  Constant3 : Constant  Value=Clm_r
  Constant4 : Constant  Value=Cnm_r
  Constant5 : Constant  Value=CL_r
  Constant6 : Constant  Value=Cmm_r
  Mux1 : Mux  Inputs=6
  delCoeff : Outport
  wires:
  Mux1/1 -> delCoeff/1
  Constant1/1 -> Mux1/1
  Constant2/1 -> Mux1/2
  Constant5/1 -> Mux1/3
  Constant3/1 -> Mux1/4
  Constant6/1 -> Mux1/5
  Constant4/1 -> Mux1/6
